simulink model "BlokDiagramSistemBis"  (R2016a)
settings: Solver=VariableStepAuto  StartTime=0.0  StopTime=10.0  RelTol=1e-3
settings Model: Creator=windows x  LastModifiedBy=windows x

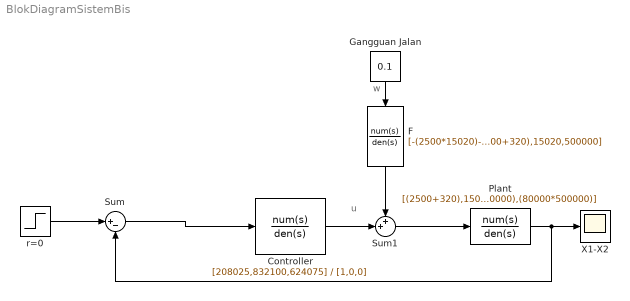
== system BlokDiagramSistemBis ==
  note: w
  note: u
  "Controller " : TransferFcn  Numerator=[208025,832100,624075]  Denominator=[1,0,0]
  F : TransferFcn  Numerator=[-(2500*15020)-(2500*500000),0,0]  Denominator=[(2500+320),15020,500000]
  Gangguan Jalan : Constant  Value=0.1
  Plant : TransferFcn  Numerator=[(2500+320),15020,500000]  Denominator=[(2500*320),(2500*(350+15020))+(320*350),(2500*(80000+500000))+(320*80000)+(350*15020),(350*500000)+(15020*80000),(80000*500000)]
  Sum : Sum  Inputs=|+-
  Sum1 : Sum  Inputs=++|
  X1-X2 : Scope
  r=0 : Step  SampleTime=0
  wires:
  r=0/1 -> Sum/1
  Sum/1 -> "Controller "/1
  "Controller "/1 -> Sum1/2
  Sum1/1 -> Plant/1
  Plant/1 -> Sum/2, X1-X2/1
  F/1 -> Sum1/1
  Gangguan Jalan/1 -> F/1
